simulink model "complementary_filter_template"  (Simulink 7.4)
settings: Solver=ode45  StartTime=0.0  StopTime=10.0  RelTol=1e-3
values from neighbouring files (symbols this model uses):
  g = 9.81    [complementary_filter_param.m]    (also in quadrocopter_param.m)
  HPF = 0.95    [complementary_filter_param.m]    (also in quadrocopter_param.m)
  LPF = 0.05    [complementary_filter_param.m]    (also in quadrocopter_param.m)
  Ts = 0.01    [complementary_filter_param.m]    (also in quadrocopter_param.m)
settings Model: Creator=Sreekanth  LastModifiedBy=Sreekanth

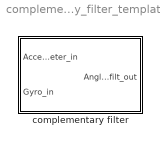
== system complementary_filter_template ==
  complementary filter : Subsystem

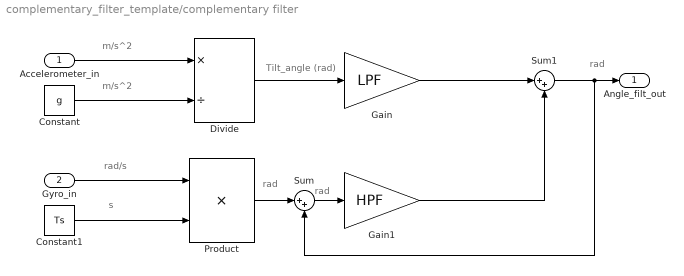
== system complementary_filter_template/complementary filter ==
  note: rad
  note: rad
  note: rad
  note: s
  note: rad/s
  note: m/s^2
  note: m/s^2
  note: Tilt_angle (rad)
  Accelerometer_in : Inport  OutDataType=fixdt(1, 16)  OutScaling=2^0
  Gyro_in : Inport  Port=2  OutDataType=fixdt(1, 16)  OutScaling=2^0
  Constant : Constant  Value=g  OutDataType=fixdt(1, 16)  OutScaling=2^0  SampleTime=Ts
  Constant1 : Constant  Value=Ts  OutDataType=fixdt(1, 16)  OutScaling=2^0  SampleTime=Ts
  Divide : Product  Inputs=*/  OutDataType=fixdt(1, 16)  OutScaling=2^-10
  Gain : Gain  Gain=LPF  ParameterDataType=fixdt(1, 16)  ParameterScaling=2^0  OutDataType=fixdt(1, 16)  OutScaling=2^0
  Gain1 : Gain  Gain=HPF  ParameterDataType=fixdt(1, 16)  ParameterScaling=2^0  OutDataType=fixdt(1, 16)  OutScaling=2^0
  Product : Product  OutDataType=fixdt(1, 16)  OutScaling=2^0  RndMeth=Zero
  Sum : Sum  Inputs=|++  OutDataType=fixdt(1, 16)  OutScaling=2^0
  Sum1 : Sum  Inputs=|++  OutDataType=fixdt(1, 16)  OutScaling=2^0
  Angle_filt_out : Outport  OutDataType=fixdt(1, 16)  OutScaling=2^0
  wires:
  Constant/1 -> Divide/2
  Accelerometer_in/1 -> Divide/1
  Gyro_in/1 -> Product/1
  Constant1/1 -> Product/2
  Sum/1 -> Gain1/1
  Sum1/1 -> Sum/2, Angle_filt_out/1
  Gain1/1 -> Sum1/2
  Gain/1 -> Sum1/1
  Product/1 -> Sum/1
  Divide/1 -> Gain/1
